simulink model "SVM"  (R2014a)
settings: Solver=ode23tb  StartTime=0.0  StopTime=0.2  RelTol=1e-3
libraries: powerlib x9, simulink x1
settings Model: Creator=ninad gaikawad  LastModifiedBy=ninad gaikawad

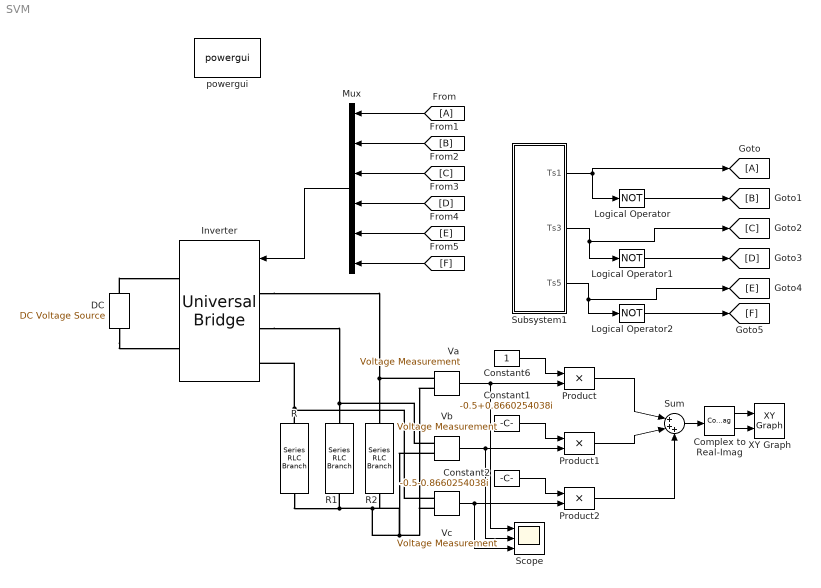
== system SVM ==
  Complex to Real-Imag : ComplexToRealImag
  Constant1 : Constant  Value=-0.5+0.8660254038i
  Constant2 : Constant  Value=-0.5-0.8660254038i
  Constant6 : Constant
  "DC " : powerlib/Electrical Sources/DC Voltage Source  Amplitude=200  Measurements=None
  Inverter : powerlib/Power Electronics/Universal Bridge  Arms=3  SnubberResistance=1e5  SnubberCapacitance=inf  Device=IGBT / Diodes  Ron=1e-3  Lon=0  ForwardVoltages="[  0  0  ]"  ForwardVoltage=0  GTOparameters=[ 10e-6 , 20e-6 ]  IGBTparameters=[ 1e-6 , 2e-6 ]  Measurements=None  Measurements_2=None  converterType=Rectifier
  Logical Operator : Logic  Operator=NOT  AllPortsSameDT=off  OutDataTypeStr=boolean
  Logical Operator1 : Logic  Operator=NOT  AllPortsSameDT=off  OutDataTypeStr=boolean
  Logical Operator2 : Logic  Operator=NOT  AllPortsSameDT=off  OutDataTypeStr=boolean
  Mux : Mux  Inputs=6
  Product : Product
  Product1 : Product
  Product2 : Product
  R : powerlib/Elements/Series RLC Branch  LConnTagsString=__new0  RConnTagsString=__new0  BranchType=R  Resistance=1000  Inductance=1e-3  SetiL0=off  InitialCurrent=0  Capacitance=1e-6  Setx0=off  InitialVoltage=0  Measurements=None
  R1 : powerlib/Elements/Series RLC Branch  LConnTagsString=__new0  RConnTagsString=__new0  BranchType=R  Resistance=1000  Inductance=1e-3  SetiL0=off  InitialCurrent=0  Capacitance=1e-6  Setx0=off  InitialVoltage=0  Measurements=None
  R2 : powerlib/Elements/Series RLC Branch  LConnTagsString=__new0  RConnTagsString=__new0  BranchType=R  Resistance=1000  Inductance=1e-3  SetiL0=off  InitialCurrent=0  Capacitance=1e-6  Setx0=off  InitialVoltage=0  Measurements=None
  Scope : Scope  NumInputPorts=3
      settings: YMin=-5~-5~-5  YMax=5~5~5
  Subsystem1 : Subsystem
  Sum : Sum  Inputs=|+++
  Va : powerlib/Measurements/Voltage Measurement  PhasorSimulation=off  OutputType=Complex  PSBequivalent=0
  Vb : powerlib/Measurements/Voltage Measurement  PhasorSimulation=off  OutputType=Complex  PSBequivalent=0
  Vc : powerlib/Measurements/Voltage Measurement  PhasorSimulation=off  OutputType=Complex  PSBequivalent=0
  XY Graph : simulink/Sinks/XY Graph  xmin=-500  xmax=500  ymin=-500  ymax=500  st=-1
  powergui : powerlib/powergui  Priority=1  SimulationMode=Continuous  SolverType=Tustin  SampleTime=50e-6  frequency=60  SPID=off  DisableSnubberDevices=off  DisableRonSwitches=off  DisableVfSwitches=off  SwTol=0  Interpol=off  DisplayEquations=off  Ts=0  methode=off  frequencyindice=0  Pbase=100e6  ErrMax=1e-4  Iterations=50  UnitsV=kV  UnitsW=MW  FunctionMessages=off  echomessages=off  HookPort=off  EnableUseOfTLC=off  x0status=blocks  RestoreLinks=warning  ResistiveCurrentMeasurement=off  Frange=[0:2:500]  Ylog=off  Xlog=on  ShowGrid=off  save=off  variable=ZData  structure=0  ZoomFFT=off  StartTime=0.0  cycles=1  DisplayStyle=1  fundamental=60  FreqAxis=off  MaxFrequency=1000  frequencyindicesteady=1  RmsSteady=1  display=off
  wires:
  Subsystem1/1(Ts1) -> Logical Operator/1, [A]
  Subsystem1/2(Ts3) -> [C], Logical Operator1/1
  Subsystem1/3(Ts5) -> [E], Logical Operator2/1
  Logical Operator/1 -> [B]
  Logical Operator1/1 -> [D]
  Logical Operator2/1 -> [F]
  [A] -> Mux/1
  [B] -> Mux/2
  [C] -> Mux/3
  [D] -> Mux/4
  [E] -> Mux/5
  [F] -> Mux/6
  Mux/1 -> Inverter/1
  Constant6/1 -> Product/1
  Va/1 -> Scope/1, Product/2
  Constant1/1 -> Product1/1
  Vb/1 -> Scope/2, Product1/2
  Constant2/1 -> Product2/1
  Product/1 -> Sum/1
  Product1/1 -> Sum/2
  Product2/1 -> Sum/3
  Sum/1 -> Complex to Real-Imag/1
  Complex to Real-Imag/1 -> XY Graph/1
  Complex to Real-Imag/2 -> XY Graph/2
  Vc/1 -> Scope/3, Product2/2
  connections:
  "DC "/RConn1 -- Inverter/RConn1
  "DC "/LConn1 -- Inverter/RConn2
  R/LConn1 -- Inverter/LConn3 -- Vc/LConn1
  Inverter/LConn2 -- Vb/LConn1 -- R1/LConn1
  Inverter/LConn1 -- Va/LConn1 -- R2/LConn1
  R/RConn1 -- R2/RConn1 -- Vb/LConn2 -- Va/LConn2 -- Vc/LConn2 -- R1/RConn1

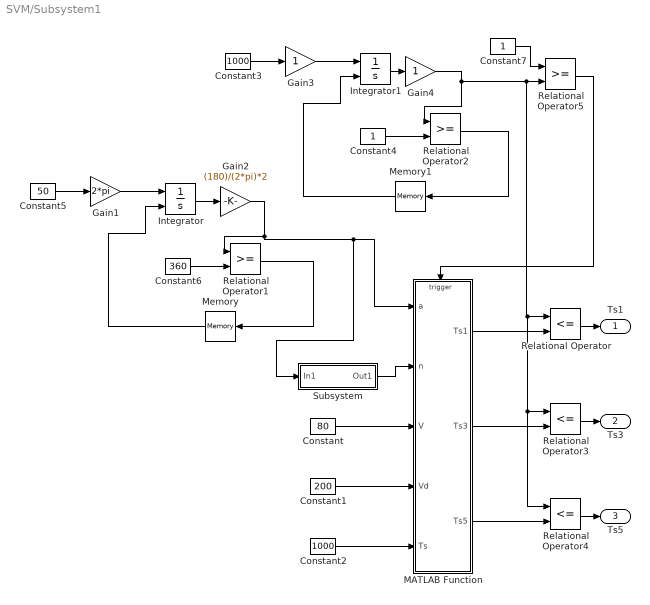
== system SVM/Subsystem1 ==
  Constant : Constant  Value=80
  Constant1 : Constant  Value=200
  Constant2 : Constant  Value=1000
  Constant3 : Constant  Value=1000
  Constant4 : Constant
  Constant5 : Constant  Value=50
  Constant6 : Constant  Value=360
  Constant7 : Constant
  Gain1 : Gain  Gain=2*pi
  Gain2 : Gain  Gain=(180)/(2*pi)*2
  Gain3 : Gain
  Gain4 : Gain
  Integrator : Integrator  ExternalReset=rising
  Integrator1 : Integrator  ExternalReset=rising
  MATLAB Function : MATLAB Function  TreatAsAtomicUnit=on
  Memory : Memory
  Memory1 : Memory
  Relational Operator : RelationalOperator  Operator=<=  OutDataTypeStr=boolean
  Relational Operator1 : RelationalOperator  OutDataTypeStr=boolean
  Relational Operator2 : RelationalOperator  OutDataTypeStr=boolean
  Relational Operator3 : RelationalOperator  Operator=<=  OutDataTypeStr=boolean
  Relational Operator4 : RelationalOperator  Operator=<=  OutDataTypeStr=boolean
  Relational Operator5 : RelationalOperator  OutDataTypeStr=boolean
  Subsystem : Subsystem
  Ts1 : Outport
  Ts3 : Outport  Port=2
  Ts5 : Outport  Port=3
  wires:
  Constant5/1 -> Gain1/1
  Constant6/1 -> Relational Operator1/2
  Gain1/1 -> Integrator/1
  Integrator/1 -> Gain2/1
  Gain2/1 -> Relational Operator1/1, Subsystem/1(In1), MATLAB Function/1(a)
  Relational Operator1/1 -> Memory/1
  Constant1/1 -> MATLAB Function/4(Vd)
  Constant/1 -> MATLAB Function/3(V)
  Subsystem/1(Out1) -> MATLAB Function/2(n)
  Gain3/1 -> Integrator1/1
  Gain4/1 -> Relational Operator4/1, Relational Operator3/1, Relational Operator/1, Relational Operator5/2, Relational Operator2/1
  Relational Operator2/1 -> Memory1/1
  Constant3/1 -> Gain3/1
  Integrator1/1 -> Gain4/1
  Constant4/1 -> Relational Operator2/2
  Constant2/1 -> MATLAB Function/5(Ts)
  MATLAB Function/3(Ts5) -> Relational Operator4/2
  Relational Operator4/1 -> Ts5/1
  Relational Operator/1 -> Ts1/1
  Relational Operator3/1 -> Ts3/1
  MATLAB Function/2(Ts3) -> Relational Operator3/2
  MATLAB Function/1(Ts1) -> Relational Operator/2
  Constant7/1 -> Relational Operator5/1
  Relational Operator5/1 -> MATLAB Function/Trigger
  Memory/1 -> Integrator/2
  Memory1/1 -> Integrator1/2

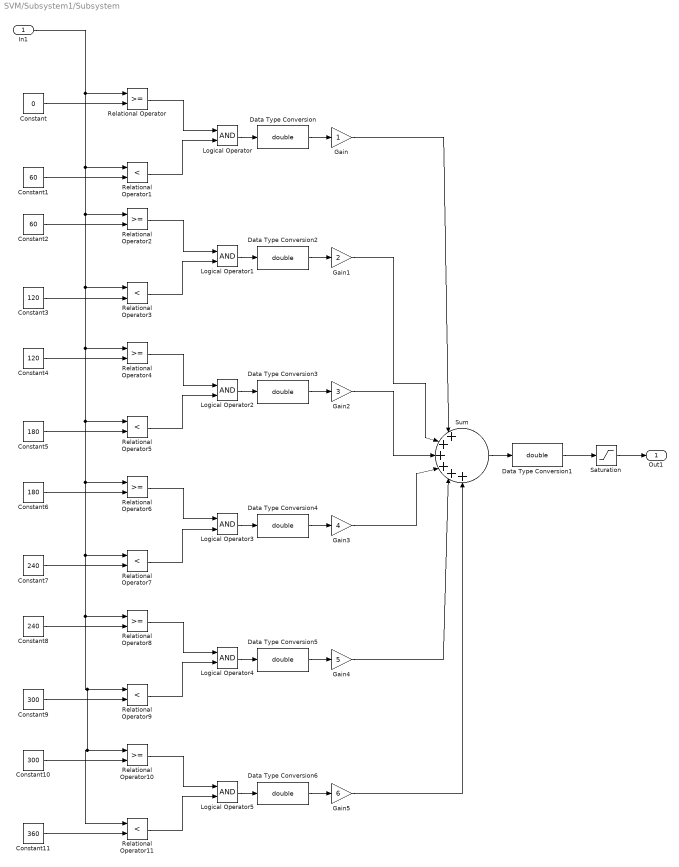
== system SVM/Subsystem1/Subsystem ==
  In1 : Inport
  Constant : Constant  Value=0
  Constant1 : Constant  Value=60
  Constant10 : Constant  Value=300
  Constant11 : Constant  Value=360
  Constant2 : Constant  Value=60
  Constant3 : Constant  Value=120
  Constant4 : Constant  Value=120
  Constant5 : Constant  Value=180
  Constant6 : Constant  Value=180
  Constant7 : Constant  Value=240
  Constant8 : Constant  Value=240
  Constant9 : Constant  Value=300
  Data Type Conversion{,1..6} (7 alike) : DataTypeConversion  OutDataTypeStr=double
  Gain : Gain
  Gain1 : Gain  Gain=2
  Gain2 : Gain  Gain=3
  Gain3 : Gain  Gain=4
  Gain4 : Gain  Gain=5
  Gain5 : Gain  Gain=6
  Logical Operator{,1..5} (6 alike) : Logic  AllPortsSameDT=off  OutDataTypeStr=boolean
  Relational Operator{,2,4,6,8,10} (6 alike) : RelationalOperator  OutDataTypeStr=boolean
  Relational Operator{1,3,5,7,9,11} (6 alike) : RelationalOperator  Operator=<  OutDataTypeStr=boolean
  Saturation : Saturate  UpperLimit=6  LowerLimit=1
  Sum : Sum  Inputs=|++++++
  Out1 : Outport
  wires:
  Constant1/1 -> Relational Operator1/2
  Constant/1 -> Relational Operator/2
  Relational Operator1/1 -> Logical Operator/2
  Relational Operator/1 -> Logical Operator/1
  Logical Operator/1 -> Data Type Conversion/1
  Data Type Conversion/1 -> Gain/1
  Gain/1 -> Sum/1
  Sum/1 -> Data Type Conversion1/1
  Data Type Conversion1/1 -> Saturation/1
  Saturation/1 -> Out1/1
  Constant3/1 -> Relational Operator3/2
  Constant2/1 -> Relational Operator2/2
  Relational Operator3/1 -> Logical Operator1/2
  Relational Operator2/1 -> Logical Operator1/1
  Logical Operator1/1 -> Data Type Conversion2/1
  Data Type Conversion2/1 -> Gain1/1
  Gain1/1 -> Sum/2
  Constant5/1 -> Relational Operator5/2
  Constant4/1 -> Relational Operator4/2
  Relational Operator5/1 -> Logical Operator2/2
  Relational Operator4/1 -> Logical Operator2/1
  Logical Operator2/1 -> Data Type Conversion3/1
  Data Type Conversion3/1 -> Gain2/1
  Gain2/1 -> Sum/3
  Constant7/1 -> Relational Operator7/2
  Constant6/1 -> Relational Operator6/2
  Relational Operator7/1 -> Logical Operator3/2
  Relational Operator6/1 -> Logical Operator3/1
  Logical Operator3/1 -> Data Type Conversion4/1
  Data Type Conversion4/1 -> Gain3/1
  Constant9/1 -> Relational Operator9/2
  Constant8/1 -> Relational Operator8/2
  Relational Operator9/1 -> Logical Operator4/2
  Relational Operator8/1 -> Logical Operator4/1
  Logical Operator4/1 -> Data Type Conversion5/1
  Data Type Conversion5/1 -> Gain4/1
  Gain4/1 -> Sum/5
  Constant11/1 -> Relational Operator11/2
  Constant10/1 -> Relational Operator10/2
  In1/1 -> Relational Operator4/1, Relational Operator11/1, Relational Operator10/1, Relational Operator9/1, Relational Operator8/1, Relational Operator7/1, Relational Operator6/1, Relational Operator5/1, Relational Operator3/1, Relational Operator2/1, Relational Operator1/1, Relational Operator/1
  Relational Operator11/1 -> Logical Operator5/2
  Relational Operator10/1 -> Logical Operator5/1
  Logical Operator5/1 -> Data Type Conversion6/1
  Data Type Conversion6/1 -> Gain5/1
  Gain5/1 -> Sum/6
  Gain3/1 -> Sum/4

== matlab function SVM/Subsystem1/MATLAB Function ==
  data: a input; Ts1 output; Ts3 output; n input; V input; Vd input; Ts input; Ts5 output
  events: trigger input RISING_EDGE_EVENT
function [Ts1,Ts3,Ts5] = fcn(a,n,V,Vd,Ts)

a=a.*pi./180;
s=(3.^0.5).*(V/Vd).*Ts;
Ta=s.*sin((n.*pi./3)-a);
Tb=s.*sin(a-(n-1).*pi./3);
To=Ts-Ta-Tb;
Ts1=0;Ts3=0;Ts5=0;
switch n
    case 1
        Ts1=(Ts-(Ta+Tb+To./2))./Ts;
        Ts3=(Ts-(Tb+To./2))./Ts;
        Ts5=(Ts-(To./2))./Ts;
    case 2
        Ts1=(Ts-(Ta+To./2))./Ts;
        Ts3=(Ts-(Ta+Tb+To./2))./Ts;
        Ts5=(Ts-(To./2))./Ts;
    case 3
        Ts1=(Ts-(To./2))./Ts;
        Ts3=(Ts-(Ta+Tb+To./2))./Ts;
        Ts5=(Ts-(Tb+To./2))./Ts;
    case 4
        Ts1=(Ts-(To./2))./Ts;
        Ts3=(Ts-(Ta+To./2))./Ts;
        Ts5=(Ts-(Ta+Tb+To./2))./Ts;
    case 5
        Ts1=(Ts-(Tb+To./2))./Ts;
        Ts3=(Ts-(To./2))./Ts;
        Ts5=(Ts-(Ta+Tb+To./2))./Ts;
    case 6
        Ts1=(Ts-(Ta+Tb+To./2))./Ts;
        Ts3=(Ts-(To./2))./Ts;
        Ts5=(Ts-(Ta+To./2))./Ts;
end
return;
